simulink model "sampleModel28"  (R2021b)
settings: Solver=VariableStepAuto  StartTime=0.0  StopTime=10.0  RelTol=1e-3
undefined symbols (not defined in the file or in its folder): DiscIntNeverNeededParam, Newton, Raphson
libraries: simulink x9
settings Model: Creator=user  LastModifiedBy=user

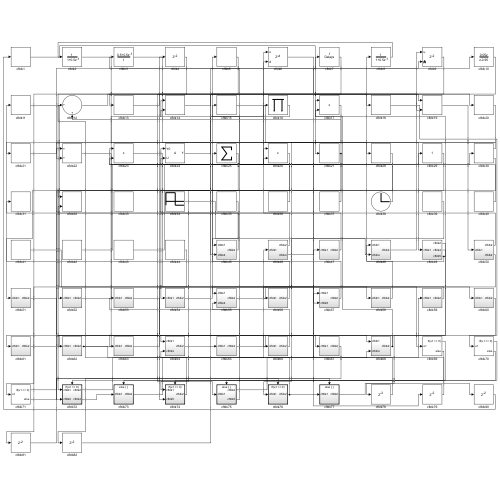
[thumbnail: Simulink's stored preview of the top-level diagram]
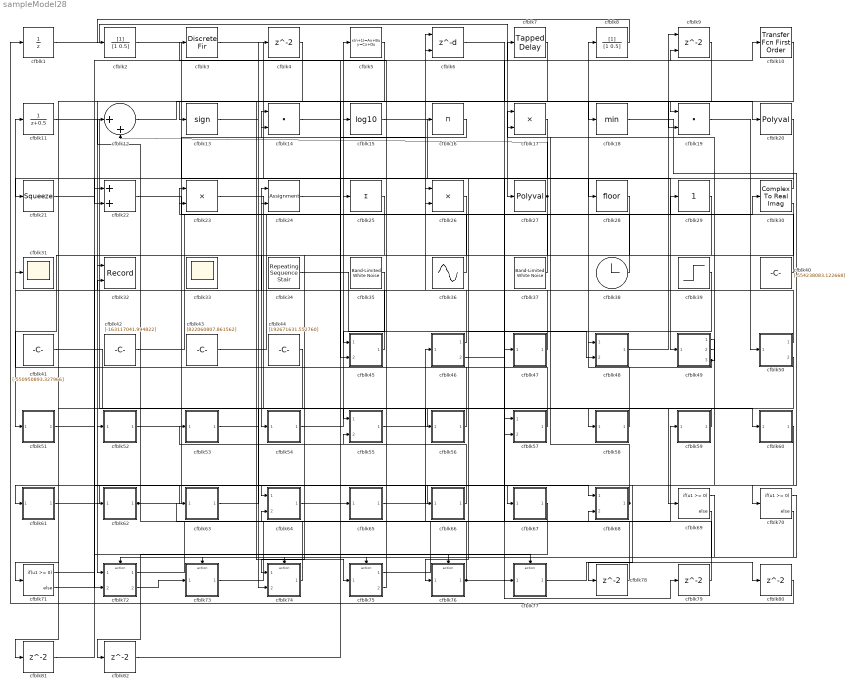
== system sampleModel28 ==
  cfblk1 : UnitDelay  HasFrameUpgradeWarning=on
  cfblk10 : simulink/Discrete/Transfer Fcn First Order  PoleZ=0.95  ICPrevOutput=0.0  DoSatur=off
  cfblk11 : DiscreteTransferFcn  SampleTime=1
  cfblk12 : Sum  Inputs=|++
  cfblk13 : Signum
  cfblk14 : DotProduct  InputSameDT=on  OutDataTypeStr=Inherit: Inherit via internal rule
  cfblk15 : Math  Operator=log10  SaturateOnIntegerOverflow=on
  cfblk16 : Product  Inputs=*
  cfblk17 : Product
  cfblk18 : MinMax
  cfblk19 : DotProduct  InputSameDT=on  OutDataTypeStr=Inherit: Inherit via internal rule
  cfblk2 : DiscreteFilter  SampleTime=1
  cfblk20 : Polyval  Coefs=[ +2.081618890e-019, -1.441693666e-014, +4.719686976e-010, -8.536869453e-006, +1.621573104e-001, -8.087801117e+001 ]
  cfblk21 : Squeeze
  cfblk22 : Sum
  cfblk23 : Product
  cfblk24 : Assignment  DiagnosticForDimensions=Warning  IndexOptions=Index vector (dialog)  Indices=1  OutputSizes=1
  cfblk25 : Sum  Inputs=+
  cfblk26 : Product  Inputs=**
  cfblk27 : Polyval  Coefs=[ +2.081618890e-019, -1.441693666e-014, +4.719686976e-010, -8.536869453e-006, +1.621573104e-001, -8.087801117e+001 ]
  cfblk28 : Rounding
  cfblk29 : simulink/Math Operations/Slider Gain  gain=1  low=0  high=2
  cfblk3 : DiscreteFir  SampleTime=1
  cfblk30 : ComplexToRealImag
  cfblk31 : Scope
  cfblk32 : Record  FileSettingsInternal="{\"entries\":[{\"content\":{\"excelSettings\":{\"content\":{},\"type\":\"Streamout.ExcelSettings\"}},\"type\":\"Streamout.FileSettingStorage\",\"uuid\":\"0d098b71-33ef-40f3-9a02-d480e724f9f5\"}],\"packageUris\":[\"http://schema.mathworks.com/mf0/streamout_blocks/R2020a\"],\"version\":\"1.0\"}"  Layout=[1 1]  SignalsInternal="{\"entries\":[{\"content\":{\"signals\":[{\"content\":{\"blockPath\":[\"sampleModel28/cfblk32\"],\"channel\":[],\"dimensions\":[1],\"domain\":\"sampleModel28/cfblk32\",\"lineColor\":\"#a2142f\",\"plots\":[1],\"port\":1,\"sid\":[\"\"],\"signalID\":1098,\"signalName\":\"cfblk5\"},\"type\":\"RecordBlkView.Signal\",\"uuid\":\"c05ac424-aba4-409f-b4c1-56cef1214d81\"},{\"content\":{\"blockPath\":[\"sampleModel28/cfblk32\"],\"channel\":[],\"dimensions\":[1],\"domain\":\"sampleModel28/cfblk32\",\"lineColor\":\"#139fff\",\"plots\":[1],\"port\":2,\"sid\":[\"\"],\"signalID\":1102,\"signalName\":\"cfblk47\"},\"type\":\"RecordBlkView.Signal\",\"uuid\":\"9ac2b13c-7aae-4351-9617-b7f3be524b82\"}]},\"type\":\"RecordBlkView.InputSignals\",\"uuid\":\"76cf4d88-b104-4784-bc6b-180bd85f36cd\"}],\"packageUris\":[\"http://schema.mathworks.com/mf0/streamout_blocks/R2020a\"],\"version\":\"1.0\"}"  VisualizationBindings="{\"xyplotplugin\":{\"info\":[{\"series\":[{\"bindingParametersList\":[{\"parameter\":\"X-Axis\",\"signalID\":1098,\"signalName\":\"cfblk5\"},{\"parameter\":\"Y-Axis\",\"signalID\":1102,\"signalName\":\"cfblk47\"}],\"seriesID\":10739}],\"subplotID\":1}]}}"  CompatibilityTag=XY
  cfblk33 : Scope
      settings: Floating=on
  cfblk34 : simulink/Sources/Repeating Sequence Stair  OutValues=[918965241.416011, -389075595.385762]  tsamp=-1  OutMin=[]  OutMax=[]  OutDataTypeStr=double  OutputDataTypeScalingMode=double  OutDataType=fixdt(0,8)  ConRadixGroup=Best Precision: Vector-wise  OutScaling=2^-12
  cfblk35 : simulink/Sources/Band-Limited White Noise  Cov=[1549154582.975929]  Ts=0.1  seed=[5555084193.000000]
  cfblk36 : Sin  Amplitude=[581087378.224464]  Bias=[-112255412.824312]  SampleTime=0
  cfblk37 : simulink/Sources/Band-Limited White Noise  Cov=[9958187217.279114]  Ts=0.1  seed=[4365866982.000000]
  cfblk38 : Clock
  cfblk39 : Step  Time=[15.000000]  Before=[-506979318.166456]  After=[921650503.309125]  SampleTime=0
  cfblk{4,78..82} (6 alike) : Delay  SampleTime=1
  cfblk40 : Constant  Value=[-554238083.122668]  SampleTime=1
  cfblk41 : Constant  Value=[-550950893.327966]  SampleTime=1
  cfblk42 : Constant  Value=[-163117041.994822]  SampleTime=1
  cfblk43 : Constant  Value=[822060807.861562]  SampleTime=1
  cfblk44 : Constant  Value=[192671631.552760]  SampleTime=1
  cfblk45 : Subsystem
  cfblk46 : Subsystem
  cfblk47 : Subsystem
  cfblk48 : Subsystem
  cfblk49 : Subsystem
  cfblk5 : DiscreteStateSpace
  cfblk50 : Subsystem
  cfblk51 : Subsystem
  cfblk52 : Subsystem
  cfblk53 : Subsystem
  cfblk54 : Subsystem
  cfblk55 : Subsystem
  cfblk56 : Subsystem
  cfblk57 : Subsystem
  cfblk58 : Subsystem
  cfblk59 : Subsystem
  cfblk6 : Delay  DelayLengthSource=Input port  SampleTime=1
      settings: InputPortMap=u0,p1
  cfblk60 : Subsystem
  cfblk61 : Subsystem
  cfblk62 : Subsystem
  cfblk63 : Subsystem
  cfblk64 : Subsystem
  cfblk65 : Subsystem
  cfblk66 : Subsystem
  cfblk67 : Subsystem
  cfblk68 : Subsystem
  cfblk69 : If  IfExpression=u1 >= 0  SampleTime=1
  cfblk7 : simulink/Discrete/Tapped Delay  vinit=0.0  samptime=-1  NumDelays=1  DelayOrder=Oldest  includeCurrent=off
  cfblk70 : If  IfExpression=u1 >= 0  SampleTime=1
  cfblk71 : If  IfExpression=u1 >= 0  SampleTime=1
  cfblk72 : Subsystem  TreatAsAtomicUnit=on
  cfblk73 : Subsystem  TreatAsAtomicUnit=on
  cfblk74 : Subsystem  TreatAsAtomicUnit=on
  cfblk75 : Subsystem  TreatAsAtomicUnit=on
  cfblk76 : Subsystem  TreatAsAtomicUnit=on
  cfblk77 : Subsystem  TreatAsAtomicUnit=on
  cfblk8 : DiscreteFilter  SampleTime=1
  cfblk9 : Delay  ShowEnablePort=on  SampleTime=1
      settings: InputPortMap=u0,e6
  wires:
  cfblk50/1(cfblk2) -> cfblk24/1
  cfblk55/1(cfblk2) -> cfblk60/1(cfblk1)
  cfblk4/1 -> cfblk75/1(cfblk1)
  cfblk1/1 -> cfblk27/1
  cfblk3/1 -> cfblk49/1(cfblk1)
  cfblk62/1(cfblk2) -> cfblk14/1, cfblk68/2(cfblk4)
  cfblk37/1 -> cfblk23/1
  cfblk58/1(cfblk2) -> cfblk8/1
  cfblk22/1 -> cfblk30/1
  cfblk38/1 -> cfblk23/2
  cfblk52/1(cfblk2) -> cfblk29/1
  cfblk2/1 -> cfblk57/2(cfblk5)
  cfblk36/1 -> cfblk6/1
  cfblk61/1(cfblk2) -> cfblk64/1(cfblk1)
  cfblk26/1 -> cfblk54/1(cfblk1)
  cfblk18/1 -> cfblk70/1
  cfblk54/1(cfblk2) -> cfblk5/1
  cfblk68/1(cfblk2) -> cfblk63/1(cfblk1), cfblk17/1
  cfblk74/1(cfblk2) -> cfblk64/2(cfblk4)
  cfblk73/1(cfblk2) -> cfblk46/1(cfblk1)
  cfblk39/1 -> cfblk76/1(cfblk1)
  cfblk65/1(cfblk2) -> cfblk67/1(cfblk1)
  cfblk29/1 -> cfblk72/1(cfblk1)
  cfblk72/1(cfblk2) -> cfblk59/1(cfblk1)
  cfblk57/1(cfblk2) -> cfblk25/1
  cfblk23/1 -> cfblk77/1(cfblk1)
  cfblk56/1(cfblk2) -> cfblk11/1
  cfblk75/1(cfblk2) -> cfblk47/1(cfblk1)
  cfblk15/1 -> cfblk28/1
  cfblk66/1(cfblk2) -> cfblk53/1(cfblk1)
  cfblk19/1 -> cfblk50/1(cfblk1)
  cfblk27/1 -> cfblk24/2, cfblk12/2, cfblk51/1(cfblk1)
  cfblk43/1 -> cfblk6/2
  cfblk41/1 -> cfblk69/1
  cfblk64/1(cfblk2) -> cfblk16/1
  cfblk49/1(cfblk2) -> cfblk62/1(cfblk1)
  cfblk35/1 -> cfblk45/1(cfblk1)
  cfblk40/1 -> cfblk15/1
  cfblk28/1 -> cfblk74/1(cfblk1)
  cfblk25/1 -> cfblk52/1(cfblk1)
  cfblk11/1 -> cfblk58/1(cfblk1)
  cfblk7/1 -> cfblk13/1
  cfblk59/1(cfblk2) -> cfblk55/1(cfblk1)
  cfblk49/2(cfblk4) -> cfblk61/1(cfblk1)
  cfblk42/1 -> cfblk4/1
  cfblk53/1(cfblk2) -> cfblk68/1(cfblk1)
  cfblk14/1 -> cfblk20/1
  cfblk48/1(cfblk2) -> cfblk9/1
  cfblk5/1 -> cfblk32/1
  cfblk30/1 -> cfblk21/1
  cfblk51/1(cfblk2) -> cfblk66/1(cfblk1)
  cfblk10/1 -> cfblk45/2(cfblk4)
  cfblk47/1(cfblk2) -> cfblk32/2
  cfblk13/1 -> cfblk19/1
  cfblk76/1(cfblk2) -> cfblk55/2(cfblk4), cfblk79/1
  cfblk49/3(cfblk5) -> cfblk48/1(cfblk1), cfblk17/2
  cfblk44/1 -> cfblk74/2(cfblk5)
  cfblk34/1 -> cfblk48/2(cfblk4)
  cfblk75/2(cfblk5) -> cfblk3/1
  cfblk30/2 -> cfblk72/2(cfblk3)
  cfblk16/1 -> cfblk14/2
  cfblk21/1 -> cfblk7/1
  cfblk45/1(cfblk2) -> cfblk31/1
  cfblk8/1 -> cfblk2/1
  cfblk17/1 -> cfblk22/2
  cfblk72/2(cfblk4) -> cfblk73/1(cfblk1)
  cfblk9/1 -> cfblk71/1
  cfblk24/1 -> cfblk10/1
  cfblk46/1(cfblk2) -> cfblk26/1
  cfblk12/1 -> cfblk18/1
  cfblk6/1 -> cfblk19/2
  cfblk46/2(cfblk4) -> cfblk9/2
  cfblk63/1(cfblk2) -> cfblk26/2
  cfblk20/1 -> cfblk56/1(cfblk1)
  cfblk69/1 -> cfblk72/Action
  cfblk69/2 -> cfblk73/Action
  cfblk70/1 -> cfblk74/Action
  cfblk70/2 -> cfblk75/Action
  cfblk71/1 -> cfblk76/Action
  cfblk71/2 -> cfblk77/Action
  cfblk60/1(cfblk2) -> cfblk78/1
  cfblk78/1 -> cfblk57/1(cfblk1)
  cfblk79/1 -> cfblk12/1
  cfblk77/1(cfblk2) -> cfblk80/1
  cfblk80/1 -> cfblk1/1
  cfblk50/2(cfblk4) -> cfblk81/1
  cfblk81/1 -> cfblk22/1
  cfblk67/1(cfblk2) -> cfblk82/1
  cfblk82/1 -> cfblk65/1(cfblk1)

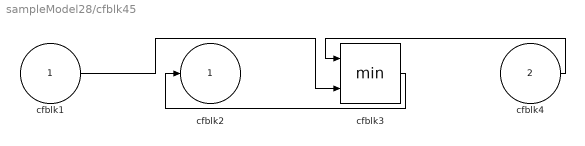
== system sampleModel28/cfblk45 ==
  cfblk1 : Inport
  cfblk4 : Inport  Port=2
  cfblk3 : MinMax  Inputs=2
  cfblk2 : Outport
  wires:
  cfblk4/1 -> cfblk3/1
  cfblk3/1 -> cfblk2/1
  cfblk1/1 -> cfblk3/2

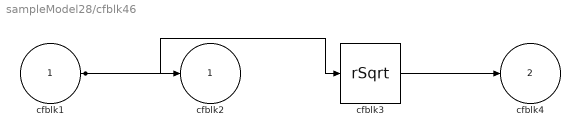
== system sampleModel28/cfblk46 ==
  cfblk1 : Inport
  cfblk3 : Sqrt  Operator=rSqrt  AlgorithmType=Newton-Raphson  SaturateOnIntegerOverflow=on
  cfblk2 : Outport
  cfblk4 : Outport  Port=2
  wires:
  cfblk3/1 -> cfblk4/1
  cfblk1/1 -> cfblk2/1, cfblk3/1

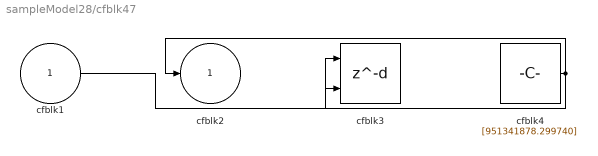
== system sampleModel28/cfblk47 ==
  cfblk1 : Inport
  cfblk3 : Delay  DelayLengthSource=Input port  SampleTime=1
      settings: InputPortMap=u0,p1
  cfblk4 : Constant  Value=[951341878.299740]  SampleTime=1
  cfblk2 : Outport
  wires:
  cfblk4/1 -> cfblk2/1, cfblk3/2
  cfblk1/1 -> cfblk3/1

== system sampleModel28/cfblk48 ==
  cfblk1 : Inport
  cfblk4 : Inport  Port=2
  cfblk3 : DiscreteIntegrator  ICPrevOutput=DiscIntNeverNeededParam  ICPrevScaledInput=DiscIntNeverNeededParam
  cfblk2 : Outport
  wires:
  cfblk1/1 -> cfblk3/1
  cfblk3/1 -> cfblk2/1

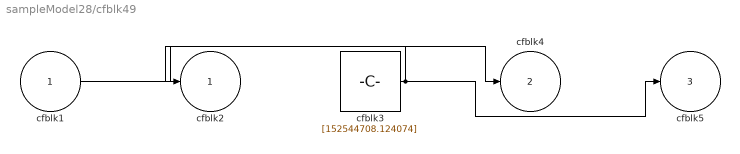
== system sampleModel28/cfblk49 ==
  cfblk1 : Inport
  cfblk3 : Constant  Value=[152544708.124074]  SampleTime=1
  cfblk2 : Outport
  cfblk4 : Outport  Port=2
  cfblk5 : Outport  Port=3
  wires:
  cfblk1/1 -> cfblk4/1
  cfblk3/1 -> cfblk5/1, cfblk2/1

== system sampleModel28/cfblk50 ==
  cfblk1 : Inport
  cfblk3 : DiscreteZeroPole  Poles=[0 0.5]  Gain=1
  cfblk2 : Outport
  cfblk4 : Outport  Port=2
  wires:
  cfblk1/1 -> cfblk3/1, cfblk2/1
  cfblk3/1 -> cfblk4/1

== system sampleModel28/cfblk51 ==
  cfblk1 : Inport
  cfblk3 : Product  Inputs=*
  cfblk2 : Outport
  wires:
  cfblk1/1 -> cfblk3/1
  cfblk3/1 -> cfblk2/1

== system sampleModel28/cfblk52 ==
  cfblk1 : Inport
  cfblk3 : Math  Operator=conj  SaturateOnIntegerOverflow=on
  cfblk4 : Squeeze
  cfblk2 : Outport
  wires:
  cfblk1/1 -> cfblk3/1
  cfblk4/1 -> cfblk2/1
  cfblk3/1 -> cfblk4/1

== system sampleModel28/cfblk53 ==
  cfblk1 : Inport
  cfblk3 : simulink/Discrete/Transfer Fcn Lead or Lag  PoleZ=0.95  ZeroZ=0.75  ICPrevOutput=0.0  ICPrevInput=0.0  DoSatur=off
      settings: SourceProductBaseCode=SL
  cfblk2 : Outport
  wires:
  cfblk1/1 -> cfblk2/1, cfblk3/1

== system sampleModel28/cfblk54 ==
  cfblk1 : Inport
  cfblk3 : DiscreteIntegrator  ICPrevOutput=DiscIntNeverNeededParam  ICPrevScaledInput=DiscIntNeverNeededParam
  cfblk4 : Constant  Value=[-26203402.256619]  SampleTime=1
  cfblk2 : Outport
  wires:
  cfblk1/1 -> cfblk3/1
  cfblk3/1 -> cfblk2/1

== system sampleModel28/cfblk55 ==
  cfblk1 : Inport
  cfblk4 : Inport  Port=2
  cfblk3 : Rounding
  cfblk2 : Outport
  wires:
  cfblk1/1 -> cfblk3/1
  cfblk4/1 -> cfblk2/1

== system sampleModel28/cfblk56 ==
  cfblk1 : Inport
  cfblk3 : Constant  Value=[-838307977.301134]  SampleTime=1
  cfblk2 : Outport
  wires:
  cfblk1/1 -> cfblk2/1

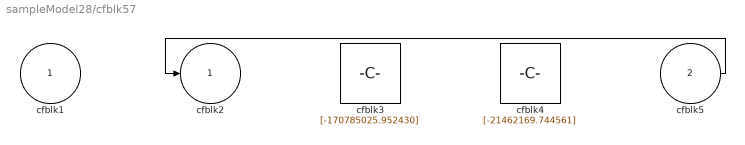
== system sampleModel28/cfblk57 ==
  cfblk1 : Inport
  cfblk5 : Inport  Port=2
  cfblk3 : Constant  Value=[-170785025.952430]  SampleTime=1
  cfblk4 : Constant  Value=[-21462169.744561]  SampleTime=1
  cfblk2 : Outport
  wires:
  cfblk5/1 -> cfblk2/1

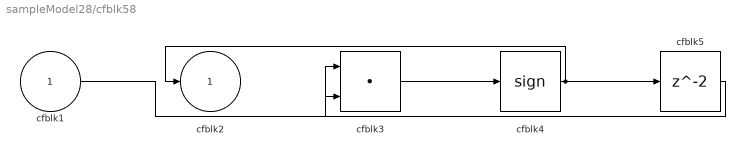
== system sampleModel28/cfblk58 ==
  cfblk1 : Inport
  cfblk3 : DotProduct  InputSameDT=on  OutDataTypeStr=Inherit: Inherit via internal rule
  cfblk4 : Signum
  cfblk5 : Delay  SampleTime=1
  cfblk2 : Outport
  wires:
  cfblk4/1 -> cfblk2/1, cfblk5/1
  cfblk1/1 -> cfblk3/1
  cfblk3/1 -> cfblk4/1
  cfblk5/1 -> cfblk3/2

== system sampleModel28/cfblk59 ==
  cfblk1 : Inport
  cfblk3 : Sum  Inputs=+-
  cfblk2 : Outport
  wires:
  cfblk1/1 -> cfblk2/1, cfblk3/1, cfblk3/2

== system sampleModel28/cfblk60 ==
  cfblk1 : Inport
  cfblk3 : Sum  Inputs=|++
  cfblk2 : Outport
  wires:
  cfblk1/1 -> cfblk3/1, cfblk3/2
  cfblk3/1 -> cfblk2/1

== system sampleModel28/cfblk61 ==
  cfblk1 : Inport
  cfblk3 : Delay  SampleTime=1
  cfblk2 : Outport
  wires:
  cfblk3/1 -> cfblk2/1
  cfblk1/1 -> cfblk3/1

== system sampleModel28/cfblk62 ==
  cfblk1 : Inport
  cfblk3 : Polyval  Coefs=[ +2.081618890e-019, -1.441693666e-014, +4.719686976e-010, -8.536869453e-006, +1.621573104e-001, -8.087801117e+001 ]
  cfblk2 : Outport
  wires:
  cfblk1/1 -> cfblk2/1, cfblk3/1

== system sampleModel28/cfblk63 ==
  cfblk1 : Inport
  cfblk3 : Bias  Bias=[-400558462.816942]
  cfblk2 : Outport
  wires:
  cfblk1/1 -> cfblk3/1
  cfblk3/1 -> cfblk2/1

== system sampleModel28/cfblk64 ==
  cfblk1 : Inport
  cfblk4 : Inport  Port=2
  cfblk3 : Delay  SampleTime=1
  cfblk2 : Outport
  wires:
  cfblk1/1 -> cfblk2/1
  cfblk4/1 -> cfblk3/1

== system sampleModel28/cfblk65 ==
  cfblk1 : Inport
  cfblk3 : Constant  Value=[637571616.540916]  SampleTime=1
  cfblk2 : Outport
  wires:
  cfblk1/1 -> cfblk2/1

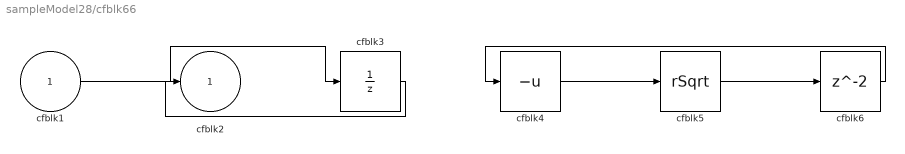
== system sampleModel28/cfblk66 ==
  cfblk1 : Inport
  cfblk3 : UnitDelay  HasFrameUpgradeWarning=on
  cfblk4 : UnaryMinus
  cfblk5 : Sqrt  Operator=rSqrt  AlgorithmType=Newton-Raphson  SaturateOnIntegerOverflow=on
  cfblk6 : Delay  SampleTime=1
  cfblk2 : Outport
  wires:
  cfblk1/1 -> cfblk3/1
  cfblk3/1 -> cfblk2/1
  cfblk4/1 -> cfblk5/1
  cfblk5/1 -> cfblk6/1
  cfblk6/1 -> cfblk4/1

== system sampleModel28/cfblk67 ==
  cfblk1 : Inport
  cfblk3 : simulink/Discrete/Transfer Fcn Real Zero  ZeroZ=0.75  ICPrevInput=0.0  DoSatur=off
      settings: SourceProductBaseCode=SL
  cfblk2 : Outport
  wires:
  cfblk1/1 -> cfblk3/1
  cfblk3/1 -> cfblk2/1

== system sampleModel28/cfblk68 ==
  cfblk1 : Inport
  cfblk4 : Inport  Port=2
  cfblk3 : Trigonometry
  cfblk2 : Outport
  wires:
  cfblk4/1 -> cfblk2/1
  cfblk1/1 -> cfblk3/1

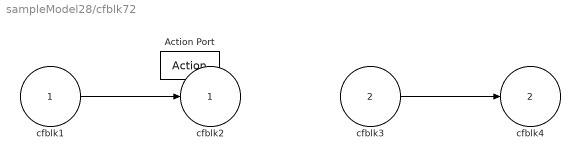
== system sampleModel28/cfblk72 ==
  cfblk1 : Inport
  cfblk3 : Inport  Port=2
  Action Port : ActionPort  ActionPortLabel=if(u1 >= 0)
  cfblk2 : Outport
  cfblk4 : Outport  Port=2
  wires:
  cfblk3/1 -> cfblk4/1
  cfblk1/1 -> cfblk2/1

== system sampleModel28/cfblk73 ==
  cfblk1 : Inport
  Action Port : ActionPort  ActionPortLabel=else
  cfblk3 : Sum  Inputs=--
  cfblk2 : Outport
  wires:
  cfblk1/1 -> cfblk3/1, cfblk3/2
  cfblk3/1 -> cfblk2/1

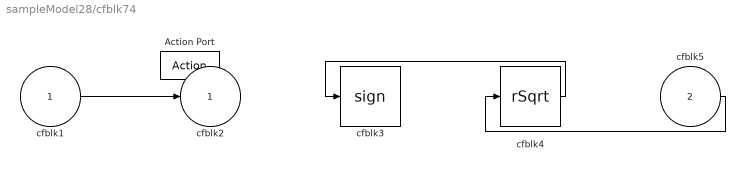
== system sampleModel28/cfblk74 ==
  cfblk1 : Inport
  cfblk5 : Inport  Port=2
  Action Port : ActionPort  ActionPortLabel=if(u1 >= 0)
  cfblk3 : Signum
  cfblk4 : Sqrt  Operator=rSqrt  AlgorithmType=Newton-Raphson  SaturateOnIntegerOverflow=on
  cfblk2 : Outport
  wires:
  cfblk1/1 -> cfblk2/1
  cfblk4/1 -> cfblk3/1
  cfblk5/1 -> cfblk4/1

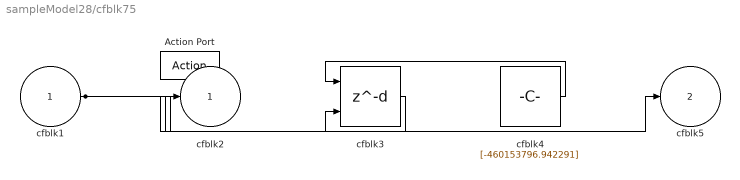
== system sampleModel28/cfblk75 ==
  cfblk1 : Inport
  Action Port : ActionPort  ActionPortLabel=else
  cfblk3 : Delay  DelayLengthSource=Input port
      settings: InputPortMap=u0,p1
  cfblk4 : Constant  Value=[-460153796.942291]  SampleTime=1
  cfblk2 : Outport
  cfblk5 : Outport  Port=2
  wires:
  cfblk1/1 -> cfblk5/1, cfblk3/2
  cfblk4/1 -> cfblk3/1
  cfblk3/1 -> cfblk2/1

== system sampleModel28/cfblk76 ==
  cfblk1 : Inport
  Action Port : ActionPort  ActionPortLabel=if(u1 >= 0)
  cfblk3 : UnaryMinus
  cfblk2 : Outport
  wires:
  cfblk1/1 -> cfblk2/1, cfblk3/1

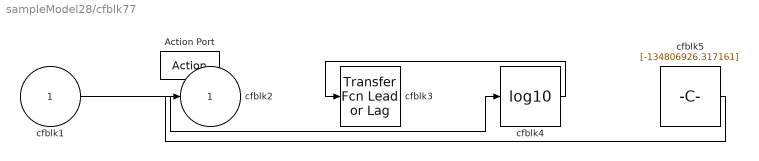
== system sampleModel28/cfblk77 ==
  cfblk1 : Inport
  Action Port : ActionPort  ActionPortLabel=else
  cfblk3 : simulink/Discrete/Transfer Fcn Lead or Lag  PoleZ=0.95  ZeroZ=0.75  ICPrevOutput=0.0  ICPrevInput=0.0  DoSatur=off
      settings: SourceProductBaseCode=SL
  cfblk4 : Math  Operator=log10  SaturateOnIntegerOverflow=on
  cfblk5 : Constant  Value=[-134806926.317161]  SampleTime=1
  cfblk2 : Outport
  wires:
  cfblk1/1 -> cfblk4/1
  cfblk5/1 -> cfblk2/1
  cfblk4/1 -> cfblk3/1
